simulink model "EvBoltCalib_Lat_v1_comb_testSteer"  (R2022b)
settings: configuration reference "ConfigSetDesktopFixedStep" (kept outside this file)
PreLoadFcn:
  | VSS_BICYCLE=Simulink.Variant('Dual=0');
  | VSS_DUAL=Simulink.Variant('Dual=1');
  | Dual=1;
model workspace (MAT data in the model file):
  Gas = 0.4
undefined symbols (not defined in the file or in its folder): AccelCmd, BattChargeLimitMaxPwr, BattChargeLimitSocBpts, BattChargeLimitTbl, BattChrgCapcty, BattDischargeLimitSocBpts, BattDischargeLimitTbl, BattDischargeMaxPwr, BattNumCellsParallel, BattNumCellsSeries, BattOpenVoltCapBpts, BattOpenVoltTbl, BattResistSocBpts, BattResistTbl, BattResistTempBpts, BrakeMaxPrs, BrakeMaxTrq, ChassisDistCg2FrontAxle, ChassisDistCg2RearAxle, ChassisVehMass, CltchCmd, DecelCmd, DiffRatio, EnvGravCnst, EnvPrs, EnvTemp, FuelSpecificGrav, GearCmd, h, InitStates, lgSw, MtrEffSpdBpts, MtrEffTbl, MtrEffTrqBpts, MtrPwrMax, MtrTrqMax, SteeringCmd, SupvsryCtrlRegenBrkCutOffTbl, SupvsryCtrlRegenSpdBpts, TestScnrioCycleNum, VEH
libraries: vehdynlibtire x8, simulink x7, vehdynlibsuspension x7, autolibutils x5, autolibshared x5, VsrLibWheel x4, vehdynlibtirecommon x3, sharedtransform x3, autolibbatterycommon x2, autolibpowerinfoutils x2, autolibsharedcoupling x2, LibPtSupervisoryCtrl x2
(part 1 of 9)
settings Model: DataDictionary=DdPassengerEv.sldd  EnableAccessToBaseWorkspace=off  SimulationMode=accelerator  PauseTimes=45  PacingRate=100000  Creator=9bt  LastModifiedBy=4qz
settings ConfigSetRef: SourceName=ConfigSetDesktopFixedStep

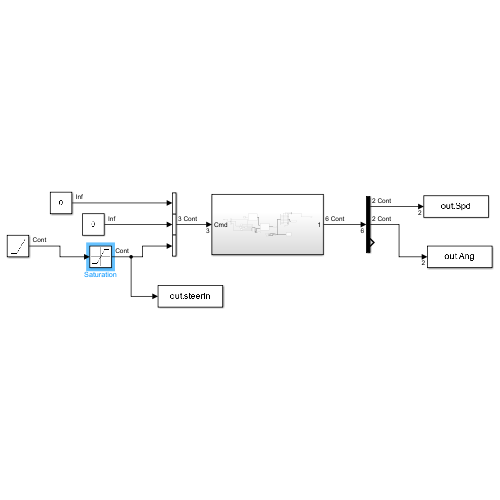
[thumbnail: Simulink's stored preview of the top-level diagram]
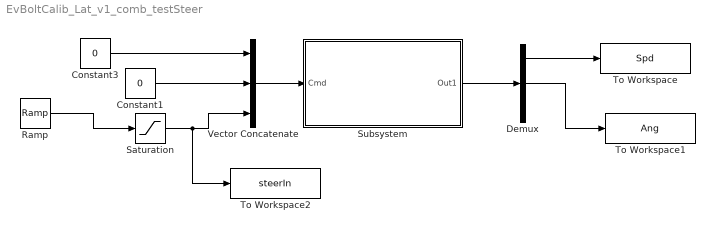
== system EvBoltCalib_Lat_v1_comb_testSteer ==
  Constant1 : Constant  Value=0
  Constant3 : Constant  Value=0
  Demux : Demux  Outputs=3
  Ramp : simulink/Sources/Ramp  slope=1  start=0  InitialOutput=0
  Saturation : Saturate  UpperLimit=2.91*pi  LowerLimit=-2.91*pi
  Subsystem : Subsystem
  To Workspace : ToWorkspace  VariableName=Spd  SampleTime=-1
      settings: Save2DSignal=2-D array (concatenate along first dimension)
  To Workspace1 : ToWorkspace  VariableName=Ang  SampleTime=-1
      settings: Save2DSignal=2-D array (concatenate along first dimension)
  To Workspace2 : ToWorkspace  VariableName=steerIn  SampleTime=-1
      settings: Save2DSignal=2-D array (concatenate along first dimension)
  Vector Concatenate : Concatenate  NumInputs=3
  wires:
  Ramp/1 -> Saturation/1
  Vector Concatenate/1 -> Subsystem/1(Cmd)
  Subsystem/1(Out1) -> Demux/1
  Constant3/1 -> Vector Concatenate/1
  Constant1/1 -> Vector Concatenate/2
  Demux/1 -> To Workspace/1
  Demux/2 -> To Workspace1/1
  Saturation/1 -> To Workspace2/1, Vector Concatenate/3

== system EvBoltCalib_Lat_v1_comb_testSteer/Subsystem ==
  Cmd : Inport
  Bus Creator : BusCreator  Inputs=AccelCmd,DecelCmd,GearCmd,CltchCmd,lgSw,SteeringCmd
  Bus Creator1 : BusCreator  Inputs=7
  Bus Creator2 : BusCreator  Inputs=2
  Bus Selector : BusSelector  OutputSignals=Veh.Chassis.VehSpd,Veh.Batt.BattSoc,Veh.Batt.BattCurr,Veh.Batt.BattVolt,Veh.Diff.Axl1.Axl1Trq,Veh.Chassis.X,Veh.Whl.WhlAngl
  Clock : Clock
  Constant : Constant  Value=0
  Constant2 : Constant
  Constant3 : Constant  Value=0
  Constant4 : Constant
  Demux : Demux  Outputs=3
  Environment : Subsystem
  Monitor : Subsystem
  To Workspace : ToWorkspace  VariableName=EvBoltCalib  SaveFormat=Structure With Time  SampleTime=-1
  Vector Concatenate : Concatenate  NumInputs=3
  Vehicle : Subsystem
  Out1 : Outport
  wires:
  Bus Creator2/1 -> Bus Selector/1, Monitor/1(Monitor)  "SimMonitor"
  Vehicle/1(Veh) -> [Veh]
  Demux/2 -> Bus Creator/2  "DecelCmd"
  [Driver] -> Bus Creator2/1  "Driver"
  Bus Selector/3 -> Bus Creator1/3  "<BattCurr>"
  Constant3/1 -> Bus Creator/4  "CltchCmd"
  Cmd/1 -> Demux/1
  Bus Creator/1 -> [Driver], Vehicle/2(Driver)
  Bus Selector/1 -> Vector Concatenate/1, Bus Creator1/1  "<VehSpd>"
  Clock/1 -> Vector Concatenate/3, Bus Creator1/7
  [Veh] -> Bus Creator2/2  "Veh"
  Bus Selector/2 -> Bus Creator1/2  "<BattSoc>"
  Bus Selector/5 -> Bus Creator1/5  "<Axl1Trq>"
  Environment/1(Env) -> Vehicle/1(Env)
  Demux/3 -> Bus Creator/6  "SteeringCmd"
  Bus Selector/4 -> Bus Creator1/4  "<BattVolt>"
  Constant/1 -> Environment/1(Grade)
  Constant4/1 -> Bus Creator/5  "lgSw"
  Bus Creator1/1 -> To Workspace/1
  Constant2/1 -> Bus Creator/3  "GearCmd"
  Demux/1 -> Bus Creator/1  "AccelCmd"
  Vector Concatenate/1 -> Out1/1
  Bus Selector/6 -> Bus Creator1/6  "<X>"
  Bus Selector/7 -> Vector Concatenate/2  "<WhlAngl>"

== system EvBoltCalib_Lat_v1_comb_testSteer/Subsystem/Environment ==
  Grade : Inport
  Friction : Constant  Value=ones(4,1).*1
  Ground Feedback : Subsystem  Variant=on  VariantControlMode=label  LabelModeActiveChoice=0
  Ground Z Level : Constant  Value=zeros(4,1)
  Subsystem : Subsystem
  Subsystem1 : Subsystem
      mask Display: disp('')
  Env : Outport
  wires:
  Subsystem/3(WindVel) -> Subsystem1/3(WindVel)
  Subsystem/2(EnvTemp) -> Subsystem1/2(EnvTemp)
  Subsystem/4(RoadGrade) -> Subsystem1/4(RoadGrade)
  Subsystem/1(EnvPrs) -> Subsystem1/1(EnvPrs)
  Subsystem1/1(Env) -> Env/1
  Friction/1 -> Ground Feedback/1(Friction)
  Ground Feedback/1(Ground) -> Subsystem1/5(GroundBus)  "Gnd"
  Ground Z Level/1 -> Ground Feedback/2(Ground Z Level)
  Grade/1 -> Subsystem/1(Grade)

== system EvBoltCalib_Lat_v1_comb_testSteer/Subsystem/Monitor ==
  Monitor : Inport
  Calculate Fuel MPG : Subsystem  Commented=on
  Calculate Powertrain Energy : Subsystem
  Terminator : Terminator
  Terminator3 : Terminator
  wires:
  Calculate Fuel MPG/1(FuelEconMPG) -> Terminator/1  "FuelEconMpg"
  Monitor/1 -> Calculate Powertrain Energy/1(Monitor), Calculate Fuel MPG/1(Monitor)
  Calculate Powertrain Energy/1(TransEnrgyOutkWh) -> Terminator3/1  "DiffEnrgyInkWh"

== system EvBoltCalib_Lat_v1_comb_testSteer/Subsystem/Vehicle ==
  Env : Inport
  Driver : Inport  Port=2
  Battery : Subsystem
  Bus Creator : BusCreator  Inputs=6
  Bus Selector : BusSelector  OutputSignals=Omega
  Front Wheel Drive : Subsystem  Variant=on  VariantControlMode=label  VariantControl=1  LabelModeActiveChoice=0
  Motor : Subsystem
  "Powertrain Supervisory Controller " : Subsystem  AncestorBlock=LibPtSupervisoryCtrl/Powertrain Supervisory Controller
      settings: LibrarySourceBlock=LibPtSupervisoryCtrl/Powertrain Supervisory Controller
  Vehicle Dynamics : Subsystem  Variant=on  VariantControlMode=label  LabelModeActiveChoice=Veh14DOF  mask{VehDynSel=Vehicle 14DOF}
      mask prompts: VehDynSel "Select the driver"
      mask init:
      | choice = get_param(gcb,'VehDynSel');
      | curBlk = gcb;
      | oldVariant = get_param(gcb,'LabelModeActiveChoice');
      | switch choice
      |     case 'Vehicle Longitudinal'
      |         set_param(curBlk, 'LabelModeActiveChoice', 'VehLong');
      | %     case 'Vehicle 3DOF'   
      | %         set_param(curBlk, 'LabelModeActiveChoice', 'Veh3DOF');
      |     case 'Vehicle 7DOF'   
      |         set_param(curBlk, 'LabelModeActiveChoice', 'Veh7DOF');
      |     case 'Vehicle 14DOF'   
      |         set_param(curBlk, 'LabelModeActiveChoice', 'Veh14DOF');
      | end
      mask TypeOptions VehDynSel: Vehicle Longitudinal | Vehicle 7DOF | Vehicle 14DOF
  Veh : Outport
  wires:
  "Powertrain Supervisory Controller "/1(SupvsryCtrl) -> Vehicle Dynamics/2(SupvsryCtrl), Motor/1(SupvsryCtrl), [SupvsryCtrl]
  Driver/1 -> "Powertrain Supervisory Controller "/1(Driver)
  Bus Creator/1 -> Veh/1  "Veh"
  [SupvsryCtrl] -> Bus Creator/1  "SupvsryCtrl"
  [Batt] -> Bus Creator/2  "Batt"
  [Mtr] -> Bus Creator/3  "Mtr"
  [Whl] -> Bus Creator/5  "Whl"
  [Chassis] -> Bus Creator/6  "Chassis"
  Battery/1(Batt) -> "Powertrain Supervisory Controller "/4(Batt), [Batt]
  Motor/1(Mtr) -> "Powertrain Supervisory Controller "/3(Mtr), [Mtr]
  Env/1 -> Vehicle Dynamics/1(Env)
  Vehicle Dynamics/2(Chassis) -> "Powertrain Supervisory Controller "/2(Chassis), [Chassis]
  Vehicle Dynamics/1(Whl) -> [Whl]
  [Whl] -> Bus Selector/1
  [Diff] -> Bus Creator/4  "Diff"
  Bus Selector/1 -> Front Wheel Drive/2(Omega)  "<Omega>"
  Front Wheel Drive/1(Diff) -> [Diff]
  Front Wheel Drive/2(AxlTrq) -> Vehicle Dynamics/3(AxlTrq)
  Front Wheel Drive/3(PropShaftSpd) -> Motor/2(MtrSpd)
  Motor/2(MtrTrq) -> Front Wheel Drive/1(DrvShfTrq)
  connections:
  Battery/RConn1 -- Motor/LConn1

== system EvBoltCalib_Lat_v1_comb_testSteer/Subsystem/Environment/Ground Feedback ==
  note: 1) Add Subsystem or Model blocks as valid variant choices.
      | 2) You cannot connect blocks at this level. At simulation, connectivity is automatically
      | determined, based on the active variant and port name matching.
  Friction : Inport
  Ground Z Level : Inport  Port=2
  3D Engine : Subsystem  VariantControl=1
  Constant : Subsystem  VariantControl=0
  Ground : Outport  VectorParamsAs1DForOutWhenUnconnected=off

== system EvBoltCalib_Lat_v1_comb_testSteer/Subsystem/Environment/Subsystem ==
  Grade : Inport
  Constant : Constant  Value=EnvPrs
  Constant1 : Constant  Value=EnvTemp
  Constant2 : Constant  Value=0
  Constant3 : Constant  Value=0
  Constant4 : Constant  Value=0
  Signal Specification : SignalSpecification  Unit=Pa
  Signal Specification1 : SignalSpecification  Unit=K
  Signal Specification2 : SignalSpecification  Unit=rad
  Signal Specification3 : SignalSpecification  Unit=m/s
  Signal Specification4 : SignalSpecification  Unit=m/s
  Signal Specification5 : SignalSpecification  Unit=m/s
  Vector Concatenate : Concatenate  NumInputs=3
  EnvPrs : Outport
  EnvTemp : Outport  Port=2
  WindVel : Outport  Port=3
  RoadGrade : Outport  Port=4
  wires:
  Constant/1 -> Signal Specification/1
  Constant2/1 -> Signal Specification3/1
  Constant1/1 -> Signal Specification1/1
  Grade/1 -> Signal Specification2/1
  Signal Specification/1 -> EnvPrs/1
  Signal Specification1/1 -> EnvTemp/1
  Signal Specification2/1 -> RoadGrade/1
  Vector Concatenate/1 -> WindVel/1
  Signal Specification3/1 -> Vector Concatenate/1  "WindX"
  Constant3/1 -> Signal Specification4/1
  Constant4/1 -> Signal Specification5/1
  Signal Specification4/1 -> Vector Concatenate/2  "WindY"
  Signal Specification5/1 -> Vector Concatenate/3  "WindZ"

== system EvBoltCalib_Lat_v1_comb_testSteer/Subsystem/Environment/Subsystem1 ==
  EnvPrs : Inport
  EnvTemp : Inport  Port=2
  WindVel : Inport  Port=3
  RoadGrade : Inport  Port=4
  GroundBus : Inport  Port=5
  Bus Creator : BusCreator  Inputs=5
  Env : Outport
  wires:
  EnvPrs/1 -> Bus Creator/1  "EnvPrs"
  EnvTemp/1 -> Bus Creator/2  "EnvTemp"
  Bus Creator/1 -> Env/1  "Env"
  WindVel/1 -> Bus Creator/3  "WindVel"
  RoadGrade/1 -> Bus Creator/4  "RoadGrade"
  GroundBus/1 -> Bus Creator/5  "GndBus"

== system EvBoltCalib_Lat_v1_comb_testSteer/Subsystem/Monitor/Calculate Fuel MPG ==
  Monitor : Inport
  Bus Selector : BusSelector  OutputSignals=Veh.Chassis.VehDist,Veh.Batt.EngPlant.FuellMassFlw
  Constant : Constant  Value=FuelSpecificGrav
  Density of Water : Gain  Gain=997
  Divide : Product  Inputs=*/
  Divide1 : Product  Inputs=*/
  Integrator : Integrator
  Saturation : Saturate  UpperLimit=inf  LowerLimit=1e-7
  Signal Specification : SignalSpecification  Unit=mi
  Signal Specification1 : SignalSpecification  Unit=m^3
  Signal Specification2 : SignalSpecification  Unit=gal
  Unit Conversion : UnitConversion
  Unit Conversion1 : UnitConversion
  FuelEconMPG : Outport
  wires:
  Divide1/1 -> FuelEconMPG/1  "FuelEconMPG"
  Divide/1 -> Signal Specification1/1
  Unit Conversion1/1 -> Signal Specification2/1
  Signal Specification2/1 -> Saturation/1
  Unit Conversion/1 -> Signal Specification/1
  Bus Selector/1 -> Unit Conversion/1  "<VehDist>"
  Bus Selector/2 -> Integrator/1  "<FuellMassFlw>"
  Integrator/1 -> Divide/1  "FuelMass"
  Density of Water/1 -> Divide/2
  Saturation/1 -> Divide1/2  "FuelVolume"
  Constant/1 -> Density of Water/1
  Signal Specification1/1 -> Unit Conversion1/1
  Monitor/1 -> Bus Selector/1
  Signal Specification/1 -> Divide1/1  "VehDistMiles"

== system EvBoltCalib_Lat_v1_comb_testSteer/Subsystem/Monitor/Calculate Powertrain Energy ==
  Monitor : Inport
  Bus Selector2 : BusSelector  OutputSignals=Veh.Diff.PwrInfo.PwrTrnsfrd.PwrTrnsfrd.PwrDriveshft
  Integrator : Integrator
  Signal Specification : SignalSpecification  Unit=J
  Signal Specification1 : SignalSpecification  Unit=kW*h
  Unit Conversion : UnitConversion
  TransEnrgyOutkWh : Outport
  wires:
  Unit Conversion/1 -> Signal Specification1/1
  Integrator/1 -> Signal Specification/1  "EnrgyTrans"
  Signal Specification/1 -> Unit Conversion/1
  Signal Specification1/1 -> TransEnrgyOutkWh/1
  Monitor/1 -> Bus Selector2/1
  Bus Selector2/1 -> Integrator/1  "<PwrDriveshft>"

== system EvBoltCalib_Lat_v1_comb_testSteer/Subsystem/Vehicle/Battery ==
  Battery : Subsystem
  Subsystem1 : Subsystem
      mask Display: disp('')
  BattOut : PMIOPort  Side=Right
  Batt : Outport
  wires:
  Battery/1(BattSoc) -> Subsystem1/1(BattSoc)
  Battery/2(BattCurr) -> Subsystem1/2(BattCurr)
  Battery/3(BattVolt) -> Subsystem1/3(BattVolt)
  Subsystem1/1(Batt) -> Batt/1
  connections:
  BattOut/RConn1 -- Battery/RConn1

== system EvBoltCalib_Lat_v1_comb_testSteer/Subsystem/Vehicle/Front Wheel Drive ==
  DrvShfTrq : Inport
  Omega : Inport  Port=2
  Ideal Diff : Subsystem  VariantControl=0
  Real Diff : Subsystem  VariantControl=1
  Diff : Outport  VectorParamsAs1DForOutWhenUnconnected=off
  AxlTrq : Outport  Port=2  VectorParamsAs1DForOutWhenUnconnected=off
  PropShaftSpd : Outport  Port=3  VectorParamsAs1DForOutWhenUnconnected=off

== system EvBoltCalib_Lat_v1_comb_testSteer/Subsystem/Vehicle/Motor ==
  SupvsryCtrl : Inport
  MtrSpd : Inport  Port=2
  Bus Creator1 : BusCreator  Inputs=1
  Bus Creator2 : BusCreator  Inputs=4
  Bus Selector1 : BusSelector  OutputSignals=Volt
  Bus Selector2 : BusSelector  OutputSignals=MtrTrqCmd
  Bus Selector3 : BusSelector  OutputSignals=PwrInfo.PwrTrnsfrd.PwrMtr,PwrInfo.PwrTrnsfrd.PwrBus
  Mapped Motor : autolibmappedmotor/Mapped Motor  port_config=Speed  param_by=Maximum torque and power  w_t=[ 0 375 750 800 ]  T_t=[0.09 0.08 0.07 0]  torque_max=MtrTrqMax  power_max=MtrPwrMax  Tc=MtrTrqTimeCnst  param_loss=Tabulated efficiency data  eff=100  w_eff=375  T_eff=0.08  Piron=0  Pbase=0  w_eff_bp=MtrEffSpdBpts.*pi/30  T_eff_bp=MtrEffTrqBpts  Temp_eff_bp=[233.15 293.15 373.15]  losses_table=[1 2;3 4]  losses_table_3d=cat(3,[1.49 1.67 2.21 3.10; 0.42 0.69 1.14 2.03; 0.06 0.24 0.78 1.68; 0.42 0.69 1.14 2.03; 1.49 1.67 2.21 3.10],[1.49 1.67 2.21 3.10; 0.42 0.69 1.14 2.03; 0.06 0.24 0.78 1.68; 0.42 0.69 1.14 2.03; 1.49 1.67 2.21 3.10],[1.49 1.67 2.21 3.10; 0.42 0.69 1.14 2.03; 0.06 0.24 0.78 1.68; 0.42 0.69 1.14 2.03; 1.49 1.67 2.21 3.10])  efficiency_table=MtrEffTbl*0.94  efficiency_table_3d=cat(3,[95 95 95 95; 95 95 95 95; 95 95 95 95; 95 95 95 95; 95 95 95 95],[95 95 95 95; 95 95 95 95; 95 95 95 95; 95 95 95 95; 95 95 95 95],[95 95 95 95; 95 95 95 95; 95 95 95 95; 95 95 95 95; 95 95 95 95])  J=5e-6  b=1e-5  omega_o=0  T_t_extended=[0 0.07 0.08 0.09 0.08 0.07 0]  w_t_extended=[-800 -750 -375 0 375 750 800]  KLossIron=0  KLossCopper=0  x_w_eff_vec=[-1047.1975511966 -942.477796076938 -837.758040957278 -733.038285837618 -628.318530717959 -523.598775598299 -418.879020478639 -314.159265358979 -285.714285713875 -209.43951023932 -104.71975511966 0 104.71975511966 209.43951023932 285.714285713875 314.159265358979 418.879020478639 523.598775598299 628.318530717959 733.038285837618 837.758040957278 942.477796076938 1047.1975511966]  x_T_eff_vec=[-360 -334.285714285714 -308.571428571429 -282.857142857143 -257.142857142857 -231.428571428571 -205.714285714286 -180 -154.285714285714 -128.571428571429 -102.857142857143 -77.1428571428572 -51.4285714285714 -25.7142857142857 0 25.7142857142857 51.4285714285714 77.1428571428572 102.857142857143 128.571428571429 154.285714285714 180 205.714285714286 231.428571428571 257.142857142857 282.857142857143 308.571428571429 334.285714285714 360]  x_tmp_eff_vec=[-0.09 -0.06 -0.03 0 0.03 0.06 0.09]  x_losses_mat=[54250.1517943165 50375.1409518653 46500.1301094142 42625.119266963 38750.1084245118 34875.0975820605 31000.0867396095 27125.0758971582 23250.065054707 19375.054212256 15500.0433698047 12629.4764797412 9803.55154311708 6774.11181875432 0 5412.5153431847 8293.80460547705 10921.9712596802 13550.1379138833 16937.6723923542 20325.2068708249 23712.7413492957 27100.2758277666 30487.8103062373 33875.3447847082 37262.879263179 40650.4137416499 44037.9482201206 47425.4826985915;44696.230836134 41503.6429192672 38311.0550024006 35118.4670855338 31925.8791686671 28733.2912518003 25540.7033349337 22348.115418067 19155.5275012002 15962.9395843336 12770.3516674669 9577.76375060014 6975.01951641212 6096.70063687888 0 4871.26380886623 6097.56206124747 8462.91205003029 11283.8827333737 14104.8534167172 16925.8241000605 19746.794783404 22567.7654667475 25388.7361500908 28209.7068334343 31030.6775167777 33851.6482001212 36672.6188834645 39493.589566808;36137.1105685043 33555.8883850397 30974.6662015752 28393.4440181105 25812.2218346459 23230.9996511813 20649.7774677168 18068.5552842522 15487.3331007875 12906.110917323 10324.8887338584 8513.56777831124 6200.01734792188 5419.28945500345 0 4330.01227454776 5420.05516555331 7522.58848891581 9220.12563933554 11525.1570491694 13830.1884590033 16135.2198688372 18440.2512786711 20745.2826885049 23050.3140983388 25355.3455081727 27660.3769180066 29965.4083278404 32270.4397376744;31619.9717474413 29361.4023369097 27102.8329263783 24844.2635158467 22585.6941053152 20327.1246947836 18068.5552842522 15809.9858737206 13551.4164631891 11292.8470526576 9034.27764212609 7449.37180602233 5425.01517943165 4741.87827312802 0 3788.76074022929 4742.54826985915 6582.26492780134 8067.6099344186 10084.5124180233 12101.4149016279 14118.3173852325 16135.2198688372 18152.1223524418 20169.0248360465 22185.9273196511 24202.8298032558 26219.7322868604 28236.6347704651;27102.8329263782 25166.9162887798 23230.9996511814 21295.0830135829 19359.1663759844 17423.249738386 15487.3331007876 13551.4164631891 11615.4998255906 9679.58318799226 8513.56777831124 6385.17583373343 4650.01301094141 4064.46709125259 0 3247.50920591082 4065.04137416498 5641.94136668686 7522.58848891582 8643.86778687709 10372.6413442524 12101.4149016279 13830.1884590033 15558.9620163787 17287.7355737541 19016.5091311295 20745.282688505 22474.0562458803 24202.8298032558;22585.6941053152 20972.4302406498 19359.1663759845 17745.9025113191 16132.6386466537 14519.3747819883 12906.110917323 11292.8470526576 9679.58318799221 8066.31932332688 7094.63981525937 5320.97986144452 3875.01084245118 3387.05590937716 0 2706.25767159235 3387.53447847082 4701.61780557238 6268.82374076318 7203.22315573091 8643.86778687704 10084.5124180232 11525.1570491694 12965.8016803156 14406.4463114618 15847.0909426079 17287.7355737541 18728.3802049003 20169.0248360465;19864.9914827262 18446.0635196743 17027.1355566225 15608.2075935706 14189.2796305187 12770.3516674668 11351.423704415 9932.4957413631 8513.56777831121 7094.63981525938 5675.71185220749 4256.78388915562 3100.00867396094 2709.64472750173 0 2165.00613727388 2710.02758277665 3761.29424445791 5015.05899261055 6268.82374076319 7522.58848891579 8776.35323706844 10030.1179852211 11283.8827333737 12537.6474815263 13791.412229679 15045.1769778316 16298.9417259842 17552.7064741369;20587.4582405459 19116.9255090783 17646.3927776108 16175.8600461432 12629.4764797412 11366.528831767 10103.581183793 8137.52276914747 6975.01951641211 5812.51626367679 4650.01301094142 3788.84294392236 2525.89529594824 2032.23354562629 0 1623.75460295541 2184.39425193603 3276.59137790406 4065.04137416499 5081.30171770625 6097.56206124746 7113.82240478872 8737.57700774416 9829.77413371214 10921.9712596802 13684.7775990372 14928.8482898587 16172.9189806802 17416.9896715018;18723.4042552922 17386.0182370571 16048.6322188219 14711.2462005868 11485.9634880614 10337.3671392553 9188.77079044916 8040.174441643 6891.57809283685 5742.98174403074 4594.38539522458 ...(+6536 chars)]  x_losses_mat_3d=[37.8947368421052 25.2631578947368 12.6315789473684 0 12 24 36;18.9473684210526 12.6315789473684 6.3157894736842 0 5.99999999999999 12 18;0 0 0 0 0 0 0;18 12 5.99999999999999 0 6.3157894736842 12.6315789473684 18.9473684210526;36 24 12 0 12.6315789473684 25.2631578947368 37.8947368421052]  CalLossMapData={}  CalLossWithTempMapData={}  aMode=aMode  RefBlkName='autolibmappedmotor/Mapped Motor'
  Memory : Memory
  Mux{,1..3} (4 alike) : Mux  Inputs=1
  Two-Way Connection1 : TwoWayConnection
  Batt : PMIOPort  Side=Left
  Mtr : Outport
  MtrTrq : Outport  Port=2
  wires:
  Mapped Motor/3 -> Mux/1, MtrTrq/1  "Trq"
  Mapped Motor/2 -> Memory/1  "Curr"
  Bus Creator1/1 -> Two-Way Connection1/1
  Mapped Motor/1 -> Bus Selector3/1
  SupvsryCtrl/1 -> Bus Selector2/1
  Two-Way Connection1/1 -> Bus Selector1/1
  Bus Selector1/1 -> Mapped Motor/1  "<Volt>"
  Bus Selector2/1 -> Mapped Motor/3  "<MtrTrqCmd>"
  Mux/1 -> Bus Creator2/2  "MtrTrq"
  Bus Creator2/1 -> Mtr/1
  Mux2/1 -> Bus Creator2/3  "MtrMechPwr"
  Bus Selector3/1 -> Mux2/1  "<PwrMtr>"
  Mux1/1 -> Bus Creator2/1  "MtrSpd"
  Bus Selector3/2 -> Mux3/1  "<PwrBus>"
  Mux3/1 -> Bus Creator2/4  "MtrElecPwr"
  Memory/1 -> Bus Creator1/1  "Curr"
  MtrSpd/1 -> Mux1/1, Mapped Motor/2
  connections:
  Batt/RConn1 -- Two-Way Connection1/RConn1

== system EvBoltCalib_Lat_v1_comb_testSteer/Subsystem/Vehicle/Powertrain Supervisory Controller  ==
  Driver : Inport
  Chassis : Inport  Port=2
  Mtr : Inport  Port=3
  Batt : Inport  Port=4
  Bus Selector : BusSelector  OutputSignals=SteeringCmd
  Engine Torque Command : Subsystem
  Subsystem1 : Subsystem
      mask Display: disp('')
  Subsystem4 : Subsystem
      mask Display: disp('')
  SupvsryCtrl : Outport
  wires:
  Engine Torque Command/4(DriverGearCmd) -> Subsystem1/4(DriverGearCmd)
  Engine Torque Command/3(BrkCmd) -> Subsystem1/3(BrkCmd)
  Engine Torque Command/2(AccelCmd) -> Subsystem1/2(AccelCmd)
  Engine Torque Command/1(MtrTrqCmd) -> Subsystem1/1(MtrTrqCmd)
  Subsystem4/6(MtrSpd) -> Engine Torque Command/6(MtrSpd)
  Subsystem4/5(BattSoc) -> Engine Torque Command/5(BattSoc)
  Subsystem4/4(VehSpd) -> Engine Torque Command/4(VehSpd)
  Subsystem4/3(DriverGearCmd) -> Engine Torque Command/3(DriverGearCmdIn)
  Mtr/1 -> Subsystem4/4(Mtr)
  Subsystem1/1(SupvsryCtrl) -> SupvsryCtrl/1
  Batt/1 -> Subsystem4/3(Batt)
  Chassis/1 -> Subsystem4/2(Chassis)
  Driver/1 -> Bus Selector/1, Subsystem4/1(Driver)
  Subsystem4/1(AccelCmd) -> Engine Torque Command/1(AccelCmdIn)
  Subsystem4/2(DecelCmd) -> Engine Torque Command/2(DecelCmdIn)
  Bus Selector/1 -> Subsystem1/5(SteeringCmd)  "<SteeringCmd>"

== system EvBoltCalib_Lat_v1_comb_testSteer/Subsystem/Vehicle/Vehicle Dynamics ==
  Env : Inport
  SupvsryCtrl : Inport  Port=2
  AxlTrq : Inport  Port=3
  Vehicle 14DOF : Subsystem  VariantControl=Veh14DOF
  Vehicle 7DOF : Subsystem  VariantControl=Veh7DOF
  Vehicle Longitudinal : Subsystem  VariantControl=VehLong
  Whl : Outport
  Chassis : Outport  Port=2

== system EvBoltCalib_Lat_v1_comb_testSteer/Subsystem/Environment/Ground Feedback/3D Engine ==
  Friction : Inport
  Ground Z Level : Inport  Port=2
  Bus Creator : BusCreator  Inputs=4
  Bus Creator2 : BusCreator  Inputs=4
  Bus Creator3 : BusCreator  Inputs=2
  Bus Selector : BusSelector  OutputSignals=HitLoc
  Data Type Conversion : DataTypeConversion  SaturateOnIntegerOverflow=off  RndMeth=Floor
  Demux : Demux
  Demux1 : Demux
  Passenger Vehicle Ray Trace Set : sim3dlib/Vehicle Terrain Sensor  Priority=1  ActorTag=SimulinkVehicle1  VehExtEn=Constant  TireRadiiExt=Constant  VehCntrLngthVal=0  TireRadiiVal=0  VehRayLngth=10  LfRayLngth=20  RfRayLngth=20  LrRayLngth=20  RrRayLngth=20  VehRayOffset=0  LfRayOffset=-1  RfRayOffset=-1  LrRayOffset=-1  RrRayOffset=-1  VehEn=on  LfEn=on  RfEn=on  LrEn=on  RrEn=on  DbgEn=off  Ts=.03  aMode=aMode
  Rate Transition : RateTransition
  Reshape10 : Reshape  OutputDimensionality=Row vector (2-D)
  Selector1 : Selector  InputPortWidth=5  IndexOptions=Index vector (dialog)  Indices=[2:5]  OutputSizes=1
  Signal Specification : SignalSpecification  Unit=m
  Signal Specification1 : SignalSpecification  Unit=1
  Terminator : Terminator
  Terminator1 : Terminator
  Terminator2 : Terminator
  Zend Select : Selector  NumberOfDimensions=2  InputPortWidth=3  IndexOptions=Select all,Index vector (dialog)  Indices=[1 3],3  OutputSizes=1,1
  Ground : Outport  VectorParamsAs1DForOutWhenUnconnected=off
  wires:
  Selector1/1 -> Rate Transition/1
  Zend Select/1 -> Reshape10/1
  Bus Selector/1 -> Zend Select/1  "<HitLoc>"
  Passenger Vehicle Ray Trace Set/2 -> Terminator1/1
  Passenger Vehicle Ray Trace Set/3 -> Terminator2/1
  Reshape10/1 -> Selector1/1
  Passenger Vehicle Ray Trace Set/1 -> Bus Selector/1
  Rate Transition/1 -> Data Type Conversion/1
  Demux/2 -> Bus Creator/2  "G_FR_z"
  Demux/1 -> Bus Creator/1  "G_FL_z"
  Demux/4 -> Bus Creator/4  "G_RR_z"
  Demux/3 -> Bus Creator/3  "G_RL_z"
  Signal Specification/1 -> Demux/1
  Signal Specification1/1 -> Demux1/1
  Demux1/1 -> Bus Creator2/1  "mu_FL"
  Bus Creator/1 -> Bus Creator3/1  "z"
  Demux1/3 -> Bus Creator2/3  "mu_RL"
  Demux1/4 -> Bus Creator2/4  "mu_RR"
  Demux1/2 -> Bus Creator2/2  "mu_FR"
  Bus Creator2/1 -> Bus Creator3/2  "mu"
  Bus Creator3/1 -> Ground/1
  Friction/1 -> Signal Specification1/1
  Data Type Conversion/1 -> Signal Specification/1
  Ground Z Level/1 -> Terminator/1

== system EvBoltCalib_Lat_v1_comb_testSteer/Subsystem/Environment/Ground Feedback/Constant ==
  Friction : Inport
  Ground Z Level : Inport  Port=2
  Bus Creator : BusCreator  Inputs=4
  Bus Creator2 : BusCreator  Inputs=4
  Bus Creator3 : BusCreator  Inputs=2
  Demux : Demux
  Demux1 : Demux
  Signal Specification : SignalSpecification  Unit=m
  Signal Specification1 : SignalSpecification  Unit=1
  Ground : Outport  VectorParamsAs1DForOutWhenUnconnected=off
  wires:
  Ground Z Level/1 -> Signal Specification/1
  Signal Specification/1 -> Demux/1
  Demux/4 -> Bus Creator/4  "G_RR_z"
  Demux/1 -> Bus Creator/1  "G_FL_z"
  Demux/3 -> Bus Creator/3  "G_RL_z"
  Demux/2 -> Bus Creator/2  "G_FR_z"
  Bus Creator/1 -> Bus Creator3/1  "z"
  Demux1/3 -> Bus Creator2/3  "mu_RL"
  Demux1/4 -> Bus Creator2/4  "mu_RR"
  Demux1/1 -> Bus Creator2/1  "mu_FL"
  Demux1/2 -> Bus Creator2/2  "mu_FR"
  Bus Creator2/1 -> Bus Creator3/2  "mu"
  Friction/1 -> Signal Specification1/1
  Signal Specification1/1 -> Demux1/1
  Bus Creator3/1 -> Ground/1

== system EvBoltCalib_Lat_v1_comb_testSteer/Subsystem/Vehicle/Battery/Battery ==
  note: Thermal model is needed to estimated battery temperature. Ambient temperture is assumed.
  Bus Creator1 : BusCreator  Inputs=1
  Bus Selector : BusSelector  OutputSignals=BattSoc
  Bus Selector2 : BusSelector  OutputSignals=Curr
  Constant : Constant  Value=EnvTemp
  Lithium Ion Battery Pack1 : Subsystem  AncestorBlock=autolibdatasheetbattery/Datasheet Battery  mask(Datasheet Battery){CapacityCtrl=Parameter, OutputVlt=Unfiltered, BattChargeMax=BattChrgCapcty, Em=BattOpenVoltTbl, CapLUTBp=BattOpenVoltCapBpts, RInt=BattResistTbl, BattTempBp=BattResistTempBpts, CapSOCBp=BattResistSocBpts, Ns=BattNumCellsSeries, Np=BattNumCellsParallel, BattCapInit=InitStates(TestScnrioCycleNum).BattSoc*BattChrgCapcty, Tc=1/1000, Vinit=3.75*72, RefBlkName='autolibdatasheetbattery/Datasheet Battery'}
      mask prompts: CapacityCtrl "autoblks:autoblkDatasheetBattery:blkPrm_CapacityCtrl"; OutputVlt "autoblks:autoblkDatasheetBattery:blkPrm_OutputVlt"; BattChargeMax "autoblks:autoblkDatasheetBattery:blkPrm_BattChargeMax"; Em "autoblks:autoblkDatasheetBattery:blkPrm_Em"; CapLUTBp "autoblks:autoblkDatasheetBattery:blkPrm_CapLUTBp"; RInt "autoblks:autoblkDatasheetBattery:blkPrm_RInt"; BattTempBp "autoblks:autoblkDatasheetBattery:blkPrm_BattTempBp"; CapSOCBp "autoblks:autoblkDatasheetBattery:blkPrm_CapSOCBp"; Ns "autoblks:autoblkDatasheetBattery:blkPrm_Ns"; Np "autoblks:autoblkDatasheetBattery:blkPrm_Np"; BattCapInit "autoblks:autoblkDatasheetBattery:blkPrm_BattCapInit"; Tc "autoblks:autoblkDatasheetBattery:blkPrm_Tc"; Vinit "autoblks:autoblkDatasheetBattery:blkPrm_Vinit"
      mask help: autoblks:autoblkDatasheetBattery:blkDesc
      mask init:
      | autoicon('autolibdatasheetbattery',gcb,'Initialization');
      settings: LibrarySourceBlock=autolibdatasheetbattery/Datasheet Battery
      mask Help: eval('autoblkshelp(''pbbatterydatasheet'')');
      mask TypeOptions CapacityCtrl: autoblks:autoblkDatasheetBattery:blkCmb_CapacityCtrlExternalInput | autoblks:autoblkDatasheetBattery:blkCmb_CapacityCtrlParameter
      mask TypeOptions OutputVlt: autoblks:autoblkDatasheetBattery:blkCmb_OutputVltFiltered | autoblks:autoblkDatasheetBattery:blkCmb_OutputVltUnfiltered
      mask DialogControl Container3 Prompt: autoblks:autoblkDatasheetBattery:blkDlg_Container3
      mask DialogControl CapacityCtrl Prompt: Initial battery capacity:
      mask DialogControl OutputVlt Prompt: Output battery voltage:
      mask DialogControl ParameterGroupVar Prompt: autoblks:autoblkDatasheetBattery:blkDlg_ParameterGroupVar
      mask DialogControl BattChargeMax Prompt: Rated capacity at nominal temperature, BattChargeMax [Ah]:
      mask DialogControl Em Prompt: Open circuit voltage table data, Em [V]:
      mask DialogControl CapLUTBp Prompt: Open circuit voltage breakpoints 1, CapLUTBp []:
      mask DialogControl RInt Prompt: Internal resistance table data, RInt [Ohms]:
      mask DialogControl BattTempBp Prompt: Battery temperature breakpoints 1, BattTempBp [K]:
      mask DialogControl CapSOCBp Prompt: Battery capacity breakpoints 2, CapSOCBp []:
      mask DialogControl Ns Prompt: Number of cells in series, Ns []:
      mask DialogControl Np Prompt: Number of cells in parallel, Np []:
      mask DialogControl BattCapInit Prompt: Initial battery capacity, BattCapInit [Ah]:
      mask DialogControl Tc Prompt: Output battery voltage time constant, Tc [s]:
      mask DialogControl Vinit Prompt: Output battery voltage initial value, Vinit [V]:
      mask Display:
      | IconInfo = autoicon('autolibdatasheetbattery', gcb, 'DrawCommands');
      | 
      | image(IconInfo.image, IconInfo.position);
      | 
      | for i = 1:numel(IconInfo.lconn)
      |     port_label('lconn', i, IconInfo.lconn{i})
      | end
      | 
      | for j = 1:numel(IconInfo.rconn)
      |     port_label('rconn', j, IconInfo.rconn{j})
      | end
      | 
      | for k = 1:numel(IconInfo.input)
      |     port_label('input', k, IconInfo.input{k})
      | end
      | 
      | for m = 1:numel(IconInfo.output)
      |     port_label('output', m, IconInfo.output{m})
      | end
  Two-Way Connection1 : TwoWayConnection
  Batt : PMIOPort  Side=Right
  BattSoc : Outport
  BattCurr : Outport  Port=2  Unit=A
  BattVolt : Outport  Port=3  Unit=V
  wires:
  Bus Selector2/1 -> Lithium Ion Battery Pack1/1(BattCurr), BattCurr/1  "<Curr>"
  Lithium Ion Battery Pack1/2(BattVolt) -> BattVolt/1, Bus Creator1/1  "Volt"
  Bus Creator1/1 -> Two-Way Connection1/1
  Constant/1 -> Lithium Ion Battery Pack1/2(BattTemp)
  Bus Selector/1 -> BattSoc/1  "<BattSoc>"
  Lithium Ion Battery Pack1/1(Info) -> Bus Selector/1
  Two-Way Connection1/1 -> Bus Selector2/1
  connections:
  Batt/RConn1 -- Two-Way Connection1/RConn1

== system EvBoltCalib_Lat_v1_comb_testSteer/Subsystem/Vehicle/Battery/Subsystem1 ==
  BattSoc : Inport
  BattCurr : Inport  Port=2
  BattVolt : Inport  Port=3
  Bus Creator : BusCreator  Inputs=3
  Batt : Outport
  wires:
  BattSoc/1 -> Bus Creator/1  "BattSoc"
  BattCurr/1 -> Bus Creator/2  "BattCurr"
  Bus Creator/1 -> Batt/1  "Batt"
  BattVolt/1 -> Bus Creator/3  "BattVolt"

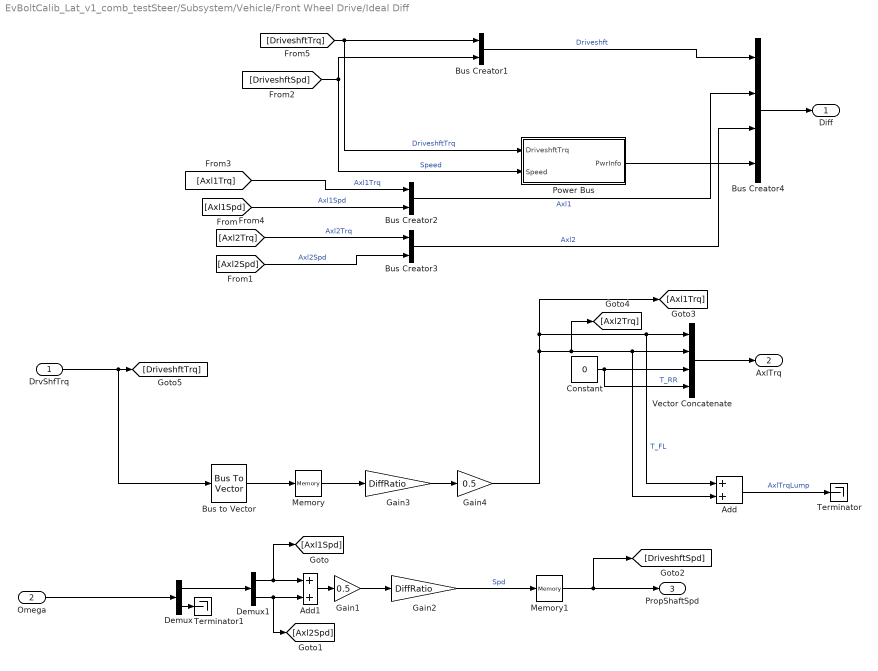
== system EvBoltCalib_Lat_v1_comb_testSteer/Subsystem/Vehicle/Front Wheel Drive/Ideal Diff ==
  DrvShfTrq : Inport
  Omega : Inport  Port=2
  Add : Sum
  Add1 : Sum
  Bus Creator1 : BusCreator  Inputs=2
  Bus Creator2 : BusCreator  Inputs=2
  Bus Creator3 : BusCreator  Inputs=2
  Bus Creator4 : BusCreator  Inputs=4
  Bus to Vector : BusToVector
  Constant : Constant  Value=0
  Demux : Demux  Outputs=[2,2]
  Demux1 : Demux  Outputs=2
  Gain1 : Gain  Gain=0.5
  Gain2 : Gain  Gain=DiffRatio
  Gain3 : Gain  Gain=DiffRatio
  Gain4 : Gain  Gain=0.5
  Memory : Memory
  Memory1 : Memory
  Power Bus : Subsystem
  Terminator : Terminator
  Terminator1 : Terminator
  Vector Concatenate : Concatenate  NumInputs=4
  Diff : Outport  VectorParamsAs1DForOutWhenUnconnected=off
  AxlTrq : Outport  Port=2  VectorParamsAs1DForOutWhenUnconnected=off
  PropShaftSpd : Outport  Port=3  VectorParamsAs1DForOutWhenUnconnected=off
  wires:
  Demux1/2 -> [Axl2Spd], Add1/2
  Vector Concatenate/1 -> AxlTrq/1
  Gain4/1 -> [Axl1Trq], Add/1, Vector Concatenate/1, [Axl2Trq], Add/2, Vector Concatenate/2  "T_FL"
  DrvShfTrq/1 -> [DriveshftTrq], Bus to Vector/1
  [DriveshftTrq] -> Power Bus/1(DriveshftTrq), Bus Creator1/1  "DriveshftTrq"
  [Axl1Spd] -> Bus Creator2/2  "Axl1Spd"
  Demux/1 -> Demux1/1
  Add1/1 -> Gain1/1
  Bus Creator4/1 -> Diff/1
  Add/1 -> Terminator/1  "AxlTrqLump"
  [Axl2Trq] -> Bus Creator3/1  "Axl2Trq"
  Omega/1 -> Demux/1
  Memory/1 -> Gain3/1
  Bus to Vector/1 -> Memory/1
  Bus Creator3/1 -> Bus Creator4/3  "Axl2"
  Bus Creator2/1 -> Bus Creator4/2  "Axl1"
  Bus Creator1/1 -> Bus Creator4/1  "Driveshft"
  [DriveshftSpd] -> Bus Creator1/2, Power Bus/2(Speed)  "Speed"
  Gain2/1 -> Memory1/1  "Spd"
  Constant/1 -> Vector Concatenate/4, Vector Concatenate/3  "T_RR"
  Demux1/1 -> [Axl1Spd], Add1/1
  Memory1/1 -> PropShaftSpd/1, [DriveshftSpd]
  Gain3/1 -> Gain4/1
  [Axl1Trq] -> Bus Creator2/1  "Axl1Trq"
  Power Bus/1(PwrInfo) -> Bus Creator4/4
  Gain1/1 -> Gain2/1
  [Axl2Spd] -> Bus Creator3/2  "Axl2Spd"
  Demux/2 -> Terminator1/1

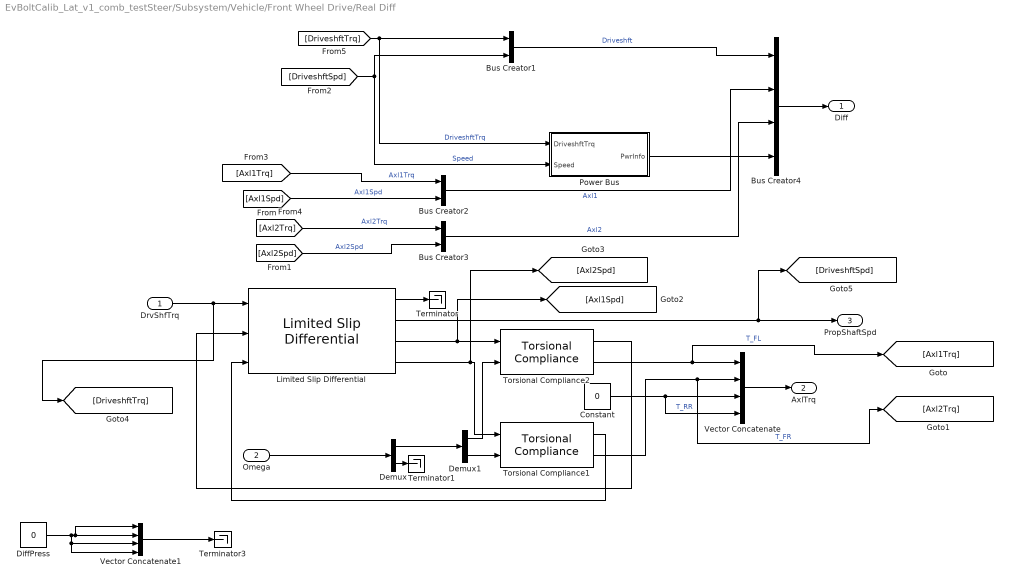
== system EvBoltCalib_Lat_v1_comb_testSteer/Subsystem/Vehicle/Front Wheel Drive/Real Diff ==
  DrvShfTrq : Inport
  Omega : Inport  Port=2
  Bus Creator1 : BusCreator  Inputs=2
  Bus Creator2 : BusCreator  Inputs=2
  Bus Creator3 : BusCreator  Inputs=2
  Bus Creator4 : BusCreator  Inputs=4
  Constant : Constant  Value=0
  Demux : Demux  Outputs=[2,2]
  Demux1 : Demux  Outputs=2
  DiffPress : Constant  Value=0
  Limited Slip Differential : autolibshareddiff/Limited Slip Differential  DiffEffModelPopup=Constant  InterpMethod=Linear point-slope  extTamb=off  shaftSwitchMask=To the left of center-line  Ndiff=7.05  Jd=0.025  bd=1e-3  Jw1=0.01  bw1=1e-3  Jw2=0.01  bw2=1e-3  omegaw1o=0  omegaw2o=0  eta=0.98  eta_tbl=reshape([0.64 0.76 0.8 0.81 0.83 0.84 0.84 0.56 0.73 0.78 0.8 0.83 0.84 0.84 0.54 0.71 0.77 0.8 0.82 0.84 0.84 0.53 0.71 0.77 0.8 0.83 0.84 0.84 0.51 0.71 0.77 0.8 0.83 0.84 0.85 0.52 0.7 0.77 0.8 0.83 0.84 0.85 0.51 0.71 0.76 0.79 0.83 0.84 0.85 0.5 0.69 0.76 0.79 0.82 0.84 0.85 0.45 0.68 0.75 0.78 0.82 0.84 0.85 0.43 0.67 0.74 0.78 0.81 0.83 0.84 0.38 0.63 0.71 0.75 0.8 0.82 0.83 0.81 0.86 0.88 0.89 0.89 0.89 0.9 0.77 0.85 0.87 0.88 0.89 0.9 0.9 0.72 0.82 0.86 0.87 0.88 0.89 0.9 0.68 0.8 0.84 0.86 0.88 0.89 0.89 0.67 0.8 0.84 0.86 0.88 0.89 0.9 0.67 0.8 0.84 0.86 0.88 0.89 0.9 0.65 0.8 0.84 0.86 0.88 0.89 0.9 0.64 0.79 0.83 0.86 0.88 0.89 0.9 0.63 0.78 0.83 0.86 0.88 0.89 0.9 0.59 0.76 0.82 0.85 0.87 0.89 0.9 0.53 0.73 0.8 0.83 0.86 0.88 0.89], 7, 11, 2)  Trq_bpts=[25, 50, 75, 100, 150, 200, 250]  omega_bpts=[52.4 78.5 105 131 157 183 209 262 314 419 524]  Temp_bpts=[290 358]  Tamb=297.15  couplingType=Pre-loaded ideal clutch  Ndisks=8  Reff=.08  Fc=1000  muc=[.16 0.13 0.115 0.11 0.105 0.1025 0.10125 .10125]  dw=[0 10 20 40 60 80 100 1000]  Tdw=[-100, -90, -50, -5, 0, 5, 50, 90, 100]  dwT=[-200, -175, -100, - 50, 0, 50, 100, 175, 200]  TTin=[-200 -175 -100 - 50 0 50 100 175 200]  Tin=[-200 -175 -100 - 50 0 50 100 175 200]  tauC=.04  IdealInterpMethod=Linear point-slope  IdealExtrapMethod=Linear  TdwInterpMethod=Flat  TdwExtrapMethod=Clip  TTinInterpMethod=Flat  TTinExtrapMethod=Clip  maxAbsSpd=5e3  aMode=2
  Power Bus : Subsystem
  Terminator : Terminator
  Terminator1 : Terminator
  Terminator3 : Terminator
  Torsional Compliance1 : autolibsharedcoupling/Torsional Compliance  port_config=Simulink  extInfo=off  k=10000  b=400  theta_o=0  domega_o=0  omega_c=300  blkID=0  aMode=2
  Torsional Compliance2 : autolibsharedcoupling/Torsional Compliance  port_config=Simulink  extInfo=off  k=10000  b=400  theta_o=0  domega_o=0  omega_c=300  blkID=0  aMode=2
  Vector Concatenate : Concatenate  NumInputs=4
  Vector Concatenate1 : Concatenate  NumInputs=4
  Diff : Outport  VectorParamsAs1DForOutWhenUnconnected=off
  AxlTrq : Outport  Port=2  VectorParamsAs1DForOutWhenUnconnected=off
  PropShaftSpd : Outport  Port=3  VectorParamsAs1DForOutWhenUnconnected=off
  wires:
  Limited Slip Differential/3 -> [Axl1Spd], Torsional Compliance2/1
  Demux1/1 -> Torsional Compliance2/2
  Limited Slip Differential/1 -> Terminator/1
  DrvShfTrq/1 -> [DriveshftTrq], Limited Slip Differential/1
  Limited Slip Differential/4 -> [Axl2Spd], Torsional Compliance1/1
  Demux1/2 -> Torsional Compliance1/2
  Demux/1 -> Demux1/1
  Torsional Compliance1/1 -> Limited Slip Differential/3
  Torsional Compliance2/1 -> Limited Slip Differential/2
  Demux/2 -> Terminator1/1
  Constant/1 -> Vector Concatenate/4, Vector Concatenate/3  "T_RR"
  Torsional Compliance1/2 -> [Axl2Trq], Vector Concatenate/2  "T_FR"
  Torsional Compliance2/2 -> [Axl1Trq], Vector Concatenate/1  "T_FL"
  Omega/1 -> Demux/1
  Vector Concatenate/1 -> AxlTrq/1
  Vector Concatenate1/1 -> Terminator3/1
  DiffPress/1 -> Vector Concatenate1/4, Vector Concatenate1/3, Vector Concatenate1/1, Vector Concatenate1/2
  [DriveshftTrq] -> Power Bus/1(DriveshftTrq), Bus Creator1/1  "DriveshftTrq"
  [Axl1Spd] -> Bus Creator2/2  "Axl1Spd"
  [Axl2Trq] -> Bus Creator3/1  "Axl2Trq"
  Bus Creator4/1 -> Diff/1
  [Axl2Spd] -> Bus Creator3/2  "Axl2Spd"
  [DriveshftSpd] -> Bus Creator1/2, Power Bus/2(Speed)  "Speed"
  Bus Creator1/1 -> Bus Creator4/1  "Driveshft"
  [Axl1Trq] -> Bus Creator2/1  "Axl1Trq"
  Power Bus/1(PwrInfo) -> Bus Creator4/4
  Bus Creator2/1 -> Bus Creator4/2  "Axl1"
  Bus Creator3/1 -> Bus Creator4/3  "Axl2"
  Limited Slip Differential/2 -> [DriveshftSpd], PropShaftSpd/1

== system EvBoltCalib_Lat_v1_comb_testSteer/Subsystem/Vehicle/Powertrain Supervisory Controller /Engine Torque Command ==
  AccelCmdIn : Inport
  DecelCmdIn : Inport  Port=2
  DriverGearCmdIn : Inport  Port=3
  VehSpd : Inport  Port=4
  BattSoc : Inport  Port=5
  MtrSpd : Inport  Port=6
  Accel Pedal to Traction Wheel Torque Request1 : Subsystem
  Battery Management System : Subsystem
  Motor Torque Arbitration and Power Management : Subsystem
  Series Regen Braking : Subsystem  InitFcn=%[~]=autosharedicon('autolibutils',gcb,0);  VariantControl=Variant
  MtrTrqCmd : Outport
  AccelCmd : Outport  Port=2
  BrkCmd : Outport  Port=3
  DriverGearCmd : Outport  Port=4
  wires:
  DecelCmdIn/1 -> Series Regen Braking/4("DecelCmd ")  "DecelPdl"
  DriverGearCmdIn/1 -> DriverGearCmd/1
  [AccelPdl] -> Motor Torque Arbitration and Power Management/2(AccelPdl)
  MtrSpd/1 -> [MotSpd], Series Regen Braking/3(MotSpd)  "MotSpd"
  AccelCmdIn/1 -> AccelCmd/1, Accel Pedal to Traction Wheel Torque Request1/1(AccelPdl), [AccelPdl]
  VehSpd/1 -> [VehSpd], Series Regen Braking/2(VehSpd)  "VehSpd"
  BattSoc/1 -> Battery Management System/1(SOC), Series Regen Braking/1(BattSoc)  "SOC"
  Battery Management System/1(BattPwrDischrgLmt) -> Motor Torque Arbitration and Power Management/3(BattPwrDisChrgLmt)  "BattPwrDischrgLmt"
  Series Regen Braking/2(" BrkCmd") -> BrkCmd/1  "BrkCmd"
  Battery Management System/2(BattPwrChrgLmt) -> Motor Torque Arbitration and Power Management/4("BattPwrChrgLmt ")  "BattPwrChrgLmt"
  Series Regen Braking/1(" MotTrqCmdRegen") -> Motor Torque Arbitration and Power Management/6(MotTrqCmdRegen)  "MotTrqCmdRegen"
  [MotSpd] -> Motor Torque Arbitration and Power Management/5(MotSpd)
  Motor Torque Arbitration and Power Management/1(MotTrqCmdFinal) -> MtrTrqCmd/1  "MotTrqCmd"
  [VehSpd] -> Accel Pedal to Traction Wheel Torque Request1/2(MotSpd)
  Accel Pedal to Traction Wheel Torque Request1/1(TrqCmd) -> Motor Torque Arbitration and Power Management/1(MotTrqCmdTrac)

== system EvBoltCalib_Lat_v1_comb_testSteer/Subsystem/Vehicle/Powertrain Supervisory Controller /Subsystem1 ==
  MtrTrqCmd : Inport
  AccelCmd : Inport  Port=2
  BrkCmd : Inport  Port=3
  DriverGearCmd : Inport  Port=4
  SteeringCmd : Inport  Port=5
  Bus Creator : BusCreator  Inputs=5
  SupvsryCtrl : Outport
  wires:
  MtrTrqCmd/1 -> Bus Creator/1  "MtrTrqCmd"
  Bus Creator/1 -> SupvsryCtrl/1  "SupvsryCtrl"
  AccelCmd/1 -> Bus Creator/2  "AccelCmd"
  BrkCmd/1 -> Bus Creator/3  "BrkCmd"
  DriverGearCmd/1 -> Bus Creator/4  "DriverGearCmd"
  SteeringCmd/1 -> Bus Creator/5  "SteeringCmd"

== system EvBoltCalib_Lat_v1_comb_testSteer/Subsystem/Vehicle/Powertrain Supervisory Controller /Subsystem4 ==
  Driver : Inport
  Chassis : Inport  Port=2
  Batt : Inport  Port=3
  Mtr : Inport  Port=4
  Bus Selector : BusSelector  OutputSignals=AccelCmd,DecelCmd,GearCmd
  Bus Selector1 : BusSelector  OutputSignals=VehSpd
  Bus Selector2 : BusSelector  OutputSignals=BattSoc
  Bus Selector3 : BusSelector  OutputSignals=MtrSpd
  AccelCmd : Outport  VectorParamsAs1DForOutWhenUnconnected=off
  DecelCmd : Outport  Port=2  VectorParamsAs1DForOutWhenUnconnected=off
  DriverGearCmd : Outport  Port=3  VectorParamsAs1DForOutWhenUnconnected=off
  VehSpd : Outport  Port=4  VectorParamsAs1DForOutWhenUnconnected=off
  BattSoc : Outport  Port=5  VectorParamsAs1DForOutWhenUnconnected=off
  MtrSpd : Outport  Port=6  VectorParamsAs1DForOutWhenUnconnected=off
  wires:
  Driver/1 -> Bus Selector/1
  Bus Selector/1 -> AccelCmd/1  "<AccelCmd>"
  Bus Selector/3 -> DriverGearCmd/1  "<GearCmd>"
  Chassis/1 -> Bus Selector1/1
  Bus Selector1/1 -> VehSpd/1  "<VehSpd>"
  Bus Selector/2 -> DecelCmd/1  "<DecelCmd>"
  Batt/1 -> Bus Selector2/1
  Bus Selector2/1 -> BattSoc/1  "<BattSoc>"
  Mtr/1 -> Bus Selector3/1
  Bus Selector3/1 -> MtrSpd/1  "<MtrSpd>"
